simulink model "sl_puma_hw5"  (R2017a)
settings: Solver=ode45  StartTime=0.0  StopTime=time(end-1)  FixedStep=.001  RelTol=1e-3  EnableMultiTasking=on
undefined symbols (not defined in the file or in its folder): time, torque
libraries: roblocks x2
settings Model: ExtModeTrigMode=oneshot  ExtModeArmWhenConnect=off  Creator=pic  LastModifiedBy=mkillpack
settings DataIOCC: SaveFormat=Array  SignalLoggingSaveFormat=ModelDataLogs  SignalLogging=off  ReturnWorkspaceOutputs=on
settings OptimizationCC: BlockReduction=off  BooleanDataType=off  ExpressionDepthLimit=2147483647  InitFltsAndDblsToZero=on  LifeSpan=inf
settings DebuggingCC: SaveWithParameterizedLinksMsg=none  UnderspecifiedInitializationDetection=Classic  MergeDetectMultiDrivingBlocksExec=none  SignalResolutionControl=TryResolveAllWithWarning  MultiTaskDSMMsg=warning  MultiTaskCondExecSysMsg=none  FcnCallInpInsideContextMsg=warning  StateNameClashWarn=warning  SFUnexpectedBacktrackingDiag=warning  SFNoUnconditionalDefaultTransitionDiag=warning  SFExecutionAtInitializationDiag=none
settings HardwareCC: ProdBitPerPointer=32  ProdBitPerSizeT=32  ProdBitPerPtrDiffT=32  ProdLargestAtomicFloat=None  ProdIntDivRoundTo=Undefined  ProdEndianess=Unspecified  ProdWordSize=32  ProdHWDeviceType=32-bit Generic  TargetUnknown=on
settings ModelReferenceCC: PropagateSignalLabelsOutOfModel=off
settings GRTTargetCC: TargetLangStandard=C89/C90 (ANSI)  ModelReferenceCompliant=off  ParMdlRefBuildCompliant=off  CompOptLevelCompliant=off  GeneratePreprocessorConditionals=Disable all  CombineOutputUpdateFcns=off  MatFileLogging=off  GRTInterface=on
settings ConfigComp: CovMetricSettings=dw  CovHtmlReporting=on  CovSaveCumulativeToWorkspaceVar=on  CovSaveSingleToWorkspaceVar=on  CovExternalEMLEnable=off  CovSFcnEnable=off

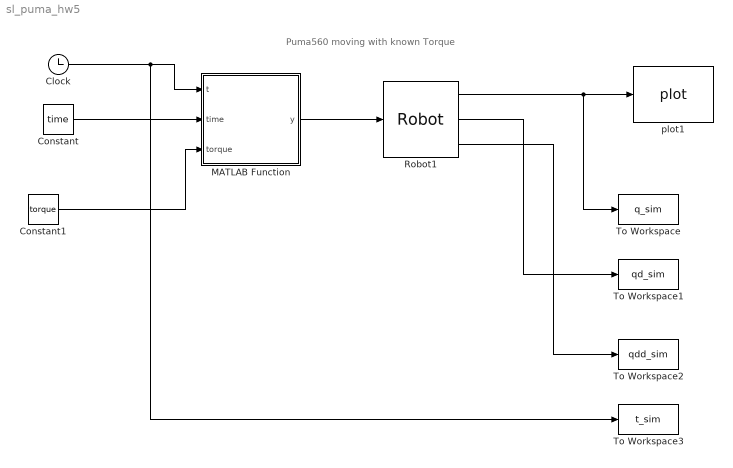
== system sl_puma_hw5 ==
  note: Puma560 moving with known Torque
  Clock : Clock
  Constant : Constant  Value=time
  Constant1 : Constant  Value=torque
  MATLAB Function : MATLAB Function  TreatAsAtomicUnit=on
  Robot1 : roblocks/Arm/Robot  robot=p560  q0=[0 0 0 0 0 0]
  To Workspace : ToWorkspace  VariableName=q_sim  SampleTime=-1
  To Workspace1 : ToWorkspace  VariableName=qd_sim  SampleTime=-1
  To Workspace2 : ToWorkspace  VariableName=qdd_sim  SampleTime=-1
  To Workspace3 : ToWorkspace  VariableName=t_sim  SampleTime=-1
  plot1 : roblocks/Arm/plot  robot=p560  fps=5  holdplot=on
  wires:
  Robot1/1 -> plot1/1, To Workspace/1
  Robot1/3 -> To Workspace2/1
  Robot1/2 -> To Workspace1/1
  Clock/1 -> To Workspace3/1, MATLAB Function/1(t)
  Constant/1 -> MATLAB Function/2(time)
  Constant1/1 -> MATLAB Function/3(torque)
  MATLAB Function/1(y) -> Robot1/1

== matlab function sl_puma_hw5/MATLAB Function ==
  data: t input; y output; time input; torque input
function y = get_torque(t, time, torque)

y = interp1(time, torque, t);

end
